simulink library "momentum_flight_control_v1"  (R2022a)
settings: Solver=VariableStepAuto  StartTime=0.0  StopTime=10.0  RelTol=1e-3
undefined symbols (not defined in the file): biasVectorConstraint_feet, Config, ConstraintMatrix_feet, DiscIntNeverNeededParam, Frames
libraries: WBToolboxLibrary x40
(part 2 of 2)

== system momentum_flight_control_v1/Flight Controller RAL-HUMANOIDS V3.0/Joint Torque Control for Flying/QP torqueControl/QP torqueControl - balancing ==
  H : Inport
  g : Inport  Port=2
  ub : Inport  Port=3
  lb : Inport  Port=4
  AEq : Inport  Port=5
  lbEq : Inport  Port=6
  ubEq : Inport  Port=7
  Enable : EnablePort
  Combine Bounds and Inequalities : MATLAB Function  TreatAsAtomicUnit=on
  MatchSignalSizes : WBToolboxLibrary/Utilities/MatchSignalSizes
      settings: SourceProductName=WholeBodyToolbox
  QP balancing-torqueControl : WBToolboxLibrary/Utilities/QP  lbA=on  ubA=on  lb=off  ub=off  computeObjVal=off  stopIfFails=off
      settings: SourceProductName=WholeBodyToolbox
  QPStatus_balancing : Outport  VectorParamsAs1DForOutWhenUnconnected=off
  QPOutput_balancing : Outport  Port=2  VectorParamsAs1DForOutWhenUnconnected=off
  wires:
  QP balancing-torqueControl/2 -> QPStatus_balancing/1
  MatchSignalSizes/1 -> QPOutput_balancing/1
  QP balancing-torqueControl/1 -> MatchSignalSizes/2
  H/1 -> QP balancing-torqueControl/1
  g/1 -> MatchSignalSizes/1, QP balancing-torqueControl/2
  AEq/1 -> Combine Bounds and Inequalities/1(AEq)
  lbEq/1 -> Combine Bounds and Inequalities/2(lbEq)
  ubEq/1 -> Combine Bounds and Inequalities/3(ubEq)
  lb/1 -> Combine Bounds and Inequalities/4(lb)
  ub/1 -> Combine Bounds and Inequalities/5(ub)
  Combine Bounds and Inequalities/1(AEq_combined) -> QP balancing-torqueControl/3
  Combine Bounds and Inequalities/2(lbEq_combined) -> QP balancing-torqueControl/4
  Combine Bounds and Inequalities/3(ubEq_combined) -> QP balancing-torqueControl/5

== system momentum_flight_control_v1/Flight Controller RAL-HUMANOIDS V3.0/Joint Torque Control for Flying/QP torqueControl/QP torqueControl - flight ==
  H : Inport
  g : Inport  Port=2
  ub : Inport  Port=3
  lb : Inport  Port=4
  Enable : EnablePort
  MatchSignalSizes : WBToolboxLibrary/Utilities/MatchSignalSizes
      settings: SourceProductName=WholeBodyToolbox
  QP flight-torqueControl : WBToolboxLibrary/Utilities/QP  lbA=off  ubA=off  lb=on  ub=on  computeObjVal=off  stopIfFails=off
      settings: SourceProductName=WholeBodyToolbox
  QPStatus_flight : Outport  VectorParamsAs1DForOutWhenUnconnected=off
  QPOutput_flight : Outport  Port=2  VectorParamsAs1DForOutWhenUnconnected=off
  wires:
  QP flight-torqueControl/2 -> QPStatus_flight/1
  lb/1 -> QP flight-torqueControl/3
  MatchSignalSizes/1 -> QPOutput_flight/1
  QP flight-torqueControl/1 -> MatchSignalSizes/2
  H/1 -> QP flight-torqueControl/1
  g/1 -> QP flight-torqueControl/2, MatchSignalSizes/1
  ub/1 -> QP flight-torqueControl/4

== system momentum_flight_control_v1/Flight Controller RAL-HUMANOIDS V3.0/Joint Torque Control for Flying/QP torqueControl/Select QP torqueControl Output ==
  QPStatus_balancing : Inport
  QPOutput_balancing : Inport  Port=2
  feetContactIsActive : Inport  Port=3
  QPStatus_flight : Inport  Port=4
  QPOutput_flight : Inport  Port=5
  Demux : Demux  Outputs=[12;Config.N_DOF]
  Switch : Switch  Criteria=u2 > Threshold  SaturateOnIntegerOverflow=off  InputSameDT=off
  Switch1 : Switch  Criteria=u2 > Threshold  SaturateOnIntegerOverflow=off  InputSameDT=off
  contactForces_QP : Terminator
  jointTorques_star : Outport  VectorParamsAs1DForOutWhenUnconnected=off
  exitFlagQP_torqueControl : Outport  Port=2  VectorParamsAs1DForOutWhenUnconnected=off
  wires:
  Switch1/1 -> jointTorques_star/1
  feetContactIsActive/1 -> Switch1/2, Switch/2
  QPStatus_balancing/1 -> Switch/1
  QPStatus_flight/1 -> Switch/3
  Switch/1 -> exitFlagQP_torqueControl/1
  QPOutput_balancing/1 -> Demux/1
  QPOutput_flight/1 -> Switch1/3
  Demux/1 -> contactForces_QP/1
  Demux/2 -> Switch1/1

== system momentum_flight_control_v1/Flight Controller RAL-HUMANOIDS V3.0/Momentum Control for Flying/QP Solver and Integrate Contact Forces Derivative/Integrate the Contact Forces Derivative ==
  contactForcesDot_star : Inport
  contactForces : Inport  Port=2
  feetContactIsActive : Inport  Port=3
  Discrete-Time Integrator1 : DiscreteIntegrator  ExternalReset=either  InitialConditionSource=external  InitialCondition=zeros(6,1)  SampleTime=Config.tStep  ICPrevOutput=DiscIntNeverNeededParam  ICPrevScaledInput=DiscIntNeverNeededParam
  Select Integrator Initial Condition : MATLAB Function  TreatAsAtomicUnit=on
  deadZone : Subsystem
  contactForces_star : Outport  VectorParamsAs1DForOutWhenUnconnected=off
  tag scope: contactForcesDot_star=global
  wires:
  Discrete-Time Integrator1/1 -> contactForces_star/1
  contactForcesDot_star/1 -> deadZone/1(u), [contactForcesDot_star]
  deadZone/1(u_cut) -> Discrete-Time Integrator1/1
  contactForces/1 -> Select Integrator Initial Condition/2(contactForces)
  feetContactIsActive/1 -> Select Integrator Initial Condition/1(feetContactIsActive), Discrete-Time Integrator1/2
  Select Integrator Initial Condition/1(contactForces_0) -> Discrete-Time Integrator1/3

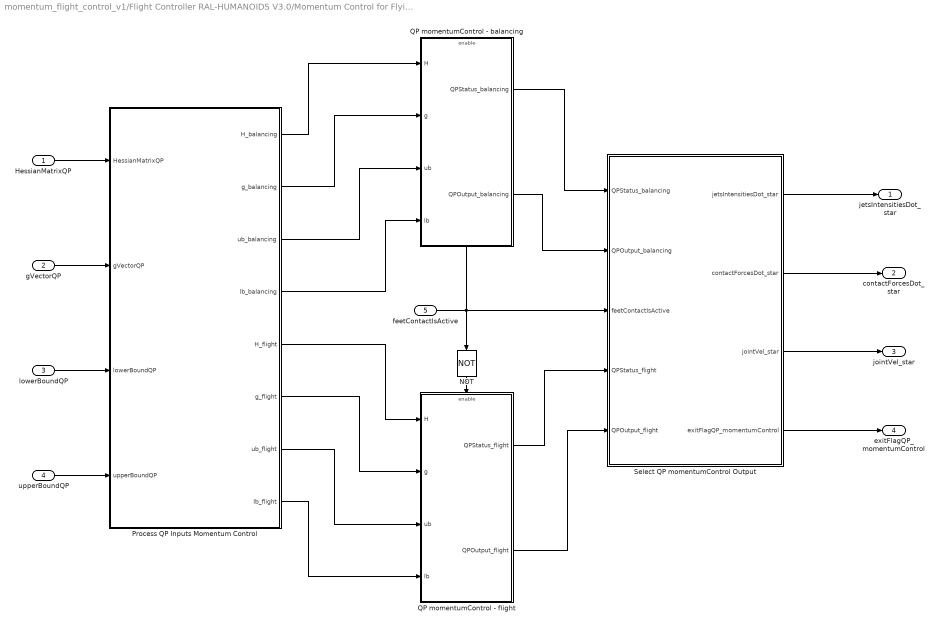
== system momentum_flight_control_v1/Flight Controller RAL-HUMANOIDS V3.0/Momentum Control for Flying/QP Solver and Integrate Contact Forces Derivative/QP momentumControl ==
  HessianMatrixQP : Inport
  gVectorQP : Inport  Port=2
  lowerBoundQP : Inport  Port=3
  upperBoundQP : Inport  Port=4
  feetContactIsActive : Inport  Port=5
  NOT : Logic  Operator=NOT  IconShape=distinctive  AllPortsSameDT=off  OutDataTypeStr=boolean
  Process QP Inputs Momentum Control : MATLAB Function  TreatAsAtomicUnit=on
  QP momentumControl - balancing : Subsystem  TreatAsAtomicUnit=on
  QP momentumControl - flight : Subsystem  TreatAsAtomicUnit=on
  Select QP momentumControl Output : Subsystem
  jetsIntensitiesDot_star : Outport  VectorParamsAs1DForOutWhenUnconnected=off
  contactForcesDot_star : Outport  Port=2  VectorParamsAs1DForOutWhenUnconnected=off
  jointVel_star : Outport  Port=3  VectorParamsAs1DForOutWhenUnconnected=off
  exitFlagQP_momentumControl : Outport  Port=4  VectorParamsAs1DForOutWhenUnconnected=off
  wires:
  gVectorQP/1 -> Process QP Inputs Momentum Control/2(gVectorQP)
  lowerBoundQP/1 -> Process QP Inputs Momentum Control/3(lowerBoundQP)
  feetContactIsActive/1 -> Select QP momentumControl Output/3(feetContactIsActive), NOT/1, QP momentumControl - balancing/Enable
  upperBoundQP/1 -> Process QP Inputs Momentum Control/4(upperBoundQP)
  HessianMatrixQP/1 -> Process QP Inputs Momentum Control/1(HessianMatrixQP)
  Select QP momentumControl Output/1(jetsIntensitiesDot_star) -> jetsIntensitiesDot_star/1
  Select QP momentumControl Output/3(jointVel_star) -> jointVel_star/1
  Select QP momentumControl Output/2(contactForcesDot_star) -> contactForcesDot_star/1
  Process QP Inputs Momentum Control/1(H_balancing) -> QP momentumControl - balancing/1(H)
  Process QP Inputs Momentum Control/2(g_balancing) -> QP momentumControl - balancing/2(g)
  Process QP Inputs Momentum Control/5(H_flight) -> QP momentumControl - flight/1(H)
  Process QP Inputs Momentum Control/6(g_flight) -> QP momentumControl - flight/2(g)
  Process QP Inputs Momentum Control/3(ub_balancing) -> QP momentumControl - balancing/3(ub)
  Process QP Inputs Momentum Control/4(lb_balancing) -> QP momentumControl - balancing/4(lb)
  Process QP Inputs Momentum Control/7(ub_flight) -> QP momentumControl - flight/3(ub)
  Process QP Inputs Momentum Control/8(lb_flight) -> QP momentumControl - flight/4(lb)
  NOT/1 -> QP momentumControl - flight/Enable
  Select QP momentumControl Output/4(exitFlagQP_momentumControl) -> exitFlagQP_momentumControl/1
  QP momentumControl - balancing/1(QPStatus_balancing) -> Select QP momentumControl Output/1(QPStatus_balancing)
  QP momentumControl - balancing/2(QPOutput_balancing) -> Select QP momentumControl Output/2(QPOutput_balancing)
  QP momentumControl - flight/1(QPStatus_flight) -> Select QP momentumControl Output/4(QPStatus_flight)
  QP momentumControl - flight/2(QPOutput_flight) -> Select QP momentumControl Output/5(QPOutput_flight)

== system momentum_flight_control_v1/Flight State Machine/Compute Gains And References/Smooth CoM and Base References/Smooth Position References ==
  smoothingTimeCoMPos : Inport
  pos_vel_acc_jerk_CoM_des : Inport  Port=2
  "CoM6D -> CoMXYZ5" : Selector  NumberOfDimensions=2  InputPortWidth=7  IndexOptions=Index vector (dialog),Index vector (dialog)  Indices=[1 2 3],[1]  OutputSizes=1,1
  Compute Smooth Jerk Reference : WBToolboxLibrary/Utilities/MinimumJerkTrajectoryGenerator  externalSettlingTime=off  settlingTime=Config.references.com.tSmoothingCoMAcc  sampleTime=Config.tStep  resetOnSettlingTime=off  firstDerivatives=on  secondDerivatives=off  explicitInitialValue=off
      settings: SourceProductName=WholeBodyToolbox
  Matrix Concatenate : Concatenate  NumInputs=4  Mode=Multidimensional array  ConcatenateDimension=2
  MinimumJerkTrajectoryGenerator : WBToolboxLibrary/Utilities/MinimumJerkTrajectoryGenerator  externalSettlingTime=on  settlingTime=3  sampleTime=Config.tStep  resetOnSettlingTime=off  firstDerivatives=on  secondDerivatives=on  explicitInitialValue=off
      settings: SourceProductName=WholeBodyToolbox
  Terminator : Terminator
  pos_vel_acc_jerk_CoM_des_smooth : Outport  VectorParamsAs1DForOutWhenUnconnected=off
  wires:
  pos_vel_acc_jerk_CoM_des/1 -> "CoM6D -> CoMXYZ5"/1
  smoothingTimeCoMPos/1 -> MinimumJerkTrajectoryGenerator/2
  MinimumJerkTrajectoryGenerator/1 -> Matrix Concatenate/1
  Matrix Concatenate/1 -> pos_vel_acc_jerk_CoM_des_smooth/1
  "CoM6D -> CoMXYZ5"/1 -> MinimumJerkTrajectoryGenerator/1
  MinimumJerkTrajectoryGenerator/2 -> Matrix Concatenate/2
  MinimumJerkTrajectoryGenerator/3 -> Matrix Concatenate/3, Compute Smooth Jerk Reference/1
  Compute Smooth Jerk Reference/1 -> Terminator/1
  Compute Smooth Jerk Reference/2 -> Matrix Concatenate/4

== system momentum_flight_control_v1/Flight State Machine/Compute Gains And References/Smooth CoM and Base References/Smooth Reference Orientations ==
  rot_vel_acc_jerk_base_des : Inport
  gainSmoothingBaseRot : Inport  Port=2
  Matrix Concatenate6 : Concatenate  NumInputs=4  Mode=Multidimensional array  ConcatenateDimension=2
  MinimumJerkTrajectoryGenerator : WBToolboxLibrary/Utilities/MinimumJerkTrajectoryGenerator  externalSettlingTime=off  settlingTime=Config.references.orientation.tSmoothingAngVel  sampleTime=Config.tStep  resetOnSettlingTime=off  firstDerivatives=on  secondDerivatives=on  explicitInitialValue=off
      settings: SourceProductName=WholeBodyToolbox
  Rotational PID Controller : Subsystem
  Selector : Selector  NumberOfDimensions=2  InputPortWidth=3  IndexOptions=Index vector (dialog),Index vector (dialog)  Indices=[1:3],[1:3]  OutputSizes=1,1
  rot_acc_vel_jerk_base_des_smooth : Outport  VectorParamsAs1DForOutWhenUnconnected=off
  wires:
  rot_vel_acc_jerk_base_des/1 -> Selector/1
  Matrix Concatenate6/1 -> rot_acc_vel_jerk_base_des_smooth/1
  Rotational PID Controller/1(w_R_b_des_smooth) -> Matrix Concatenate6/1
  Rotational PID Controller/2(body_omega_b_des_smooth) -> MinimumJerkTrajectoryGenerator/1
  MinimumJerkTrajectoryGenerator/1 -> Matrix Concatenate6/2
  MinimumJerkTrajectoryGenerator/2 -> Matrix Concatenate6/3
  Selector/1 -> Rotational PID Controller/1(w_R_b_des)
  gainSmoothingBaseRot/1 -> Rotational PID Controller/2(gainSmoothingBaseRot)
  MinimumJerkTrajectoryGenerator/3 -> Matrix Concatenate6/4

== system momentum_flight_control_v1/Flight Controller RAL-HUMANOIDS V3.0/Momentum Control for Flying/QP Solver and Integrate Contact Forces Derivative/Integrate the Contact Forces Derivative/deadZone ==
  u : Inport
  Constant : Constant  Value=Config.sat.deadZoneThreshold
  Deadzone Function : MATLAB Function  TreatAsAtomicUnit=on
  u_cut : Outport  VectorParamsAs1DForOutWhenUnconnected=off
  wires:
  Deadzone Function/1(y) -> u_cut/1
  u/1 -> Deadzone Function/1(u)
  Constant/1 -> Deadzone Function/2(thr)

== system momentum_flight_control_v1/Flight Controller RAL-HUMANOIDS V3.0/Momentum Control for Flying/QP Solver and Integrate Contact Forces Derivative/QP momentumControl/QP momentumControl - balancing ==
  H : Inport
  g : Inport  Port=2
  ub : Inport  Port=3
  lb : Inport  Port=4
  Enable : EnablePort
  MatchSignalSizes : WBToolboxLibrary/Utilities/MatchSignalSizes
      settings: SourceProductName=WholeBodyToolbox
  QP balancing-momentumControl : WBToolboxLibrary/Utilities/QP  lbA=off  ubA=off  lb=on  ub=on  computeObjVal=off  stopIfFails=off
      settings: SourceProductName=WholeBodyToolbox
  QPStatus_balancing : Outport  VectorParamsAs1DForOutWhenUnconnected=off
  QPOutput_balancing : Outport  Port=2  VectorParamsAs1DForOutWhenUnconnected=off
  wires:
  QP balancing-momentumControl/2 -> QPStatus_balancing/1
  lb/1 -> QP balancing-momentumControl/3
  MatchSignalSizes/1 -> QPOutput_balancing/1
  QP balancing-momentumControl/1 -> MatchSignalSizes/2
  H/1 -> QP balancing-momentumControl/1
  g/1 -> QP balancing-momentumControl/2, MatchSignalSizes/1
  ub/1 -> QP balancing-momentumControl/4

== system momentum_flight_control_v1/Flight Controller RAL-HUMANOIDS V3.0/Momentum Control for Flying/QP Solver and Integrate Contact Forces Derivative/QP momentumControl/QP momentumControl - flight ==
  H : Inport
  g : Inport  Port=2
  ub : Inport  Port=3
  lb : Inport  Port=4
  Enable : EnablePort
  MatchSignalSizes : WBToolboxLibrary/Utilities/MatchSignalSizes
      settings: SourceProductName=WholeBodyToolbox
  QP flight-momentumControl : WBToolboxLibrary/Utilities/QP  lbA=off  ubA=off  lb=on  ub=on  computeObjVal=off  stopIfFails=off
      settings: SourceProductName=WholeBodyToolbox
  QPStatus_flight : Outport  VectorParamsAs1DForOutWhenUnconnected=off
  QPOutput_flight : Outport  Port=2  VectorParamsAs1DForOutWhenUnconnected=off
  wires:
  QP flight-momentumControl/2 -> QPStatus_flight/1
  lb/1 -> QP flight-momentumControl/3
  MatchSignalSizes/1 -> QPOutput_flight/1
  QP flight-momentumControl/1 -> MatchSignalSizes/2
  H/1 -> QP flight-momentumControl/1
  g/1 -> QP flight-momentumControl/2, MatchSignalSizes/1
  ub/1 -> QP flight-momentumControl/4

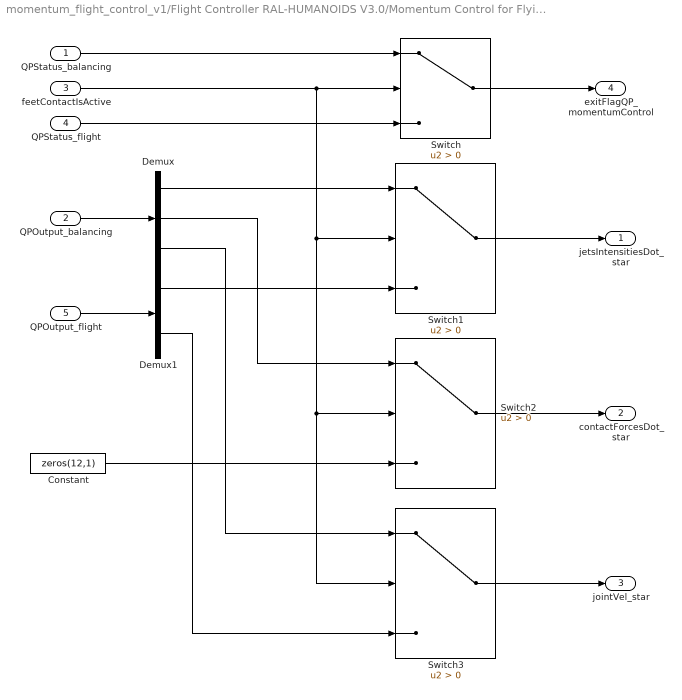
== system momentum_flight_control_v1/Flight Controller RAL-HUMANOIDS V3.0/Momentum Control for Flying/QP Solver and Integrate Contact Forces Derivative/QP momentumControl/Select QP momentumControl Output ==
  QPStatus_balancing : Inport
  QPOutput_balancing : Inport  Port=2
  feetContactIsActive : Inport  Port=3
  QPStatus_flight : Inport  Port=4
  QPOutput_flight : Inport  Port=5
  Constant : Constant  Value=zeros(12,1)
  Demux : Demux  Outputs=[4;12;Config.N_DOF]
  Demux1 : Demux  Outputs=[4;Config.N_DOF]
  Switch{,1..3} (4 alike) : Switch  Criteria=u2 > Threshold  SaturateOnIntegerOverflow=off  InputSameDT=off
  jetsIntensitiesDot_star : Outport  VectorParamsAs1DForOutWhenUnconnected=off
  contactForcesDot_star : Outport  Port=2  VectorParamsAs1DForOutWhenUnconnected=off
  jointVel_star : Outport  Port=3  VectorParamsAs1DForOutWhenUnconnected=off
  exitFlagQP_momentumControl : Outport  Port=4  VectorParamsAs1DForOutWhenUnconnected=off
  wires:
  Switch2/1 -> contactForcesDot_star/1
  Switch1/1 -> jetsIntensitiesDot_star/1
  Switch3/1 -> jointVel_star/1
  feetContactIsActive/1 -> Switch3/2, Switch2/2, Switch1/2, Switch/2
  QPStatus_balancing/1 -> Switch/1
  QPStatus_flight/1 -> Switch/3
  Switch/1 -> exitFlagQP_momentumControl/1
  QPOutput_balancing/1 -> Demux/1
  QPOutput_flight/1 -> Demux1/1
  Demux/1 -> Switch1/1
  Demux1/1 -> Switch1/3
  Demux/2 -> Switch2/1
  Constant/1 -> Switch2/3
  Demux/3 -> Switch3/1
  Demux1/2 -> Switch3/3

== system momentum_flight_control_v1/Flight State Machine/Compute Gains And References/Smooth CoM and Base References/Smooth Reference Orientations/Rotational PID Controller ==
  w_R_b_des : Inport
  gainSmoothingBaseRot : Inport  Port=2
  Compute Rotation Matrix Derivative : MATLAB Function  TreatAsAtomicUnit=on
  Discrete-Time Integrator2 : DiscreteIntegrator  InitialConditionSource=external  InitialCondition=zeros(3,1)  SampleTime=Config.tStep  ICPrevOutput=DiscIntNeverNeededParam  ICPrevScaledInput=DiscIntNeverNeededParam
  "holder " : WBToolboxLibrary/Utilities/holder 
      settings: SourceProductName=WholeBodyToolbox
  w_R_b_des_smooth : Outport  VectorParamsAs1DForOutWhenUnconnected=off
  body_omega_b_des_smooth : Outport  Port=2  VectorParamsAs1DForOutWhenUnconnected=off
  wires:
  "holder "/1 -> Discrete-Time Integrator2/2
  Compute Rotation Matrix Derivative/2(RDot) -> Discrete-Time Integrator2/1
  Discrete-Time Integrator2/1 -> w_R_b_des_smooth/1, Compute Rotation Matrix Derivative/3(w_R_b)
  w_R_b_des/1 -> "holder "/1, Compute Rotation Matrix Derivative/2(w_R_b_des)
  Compute Rotation Matrix Derivative/1(b_omega_b) -> body_omega_b_des_smooth/1
  gainSmoothingBaseRot/1 -> Compute Rotation Matrix Derivative/1(gainSmoothingBaseRot)

== matlab function momentum_flight_control_v1/Get System State/fromPosRPYtoTransfMatrix ==
  data: pos_rpy input; w_H_b output
function w_H_b = fromPosRpyToTransfMatrixFCN(pos_rpy)

    w_H_b = wbc.fromPosRpyToTransfMatrix(pos_rpy);
end

== matlab function momentum_flight_control_v1/Flight Controller RAL-HUMANOIDS V3.0/Joint Torque Control for Flying/QP torqueControl/Process QP Inputs Torque Control ==
  data: HessianMatrixQP input; H_balancing output; gVectorQP input; InequalityConstrMatrix input; biasVectorInequalityConstr input; g_balancing output; ub_balancing output; lb_balancing output; Aeq_balancing output; lbEq_balancing output; ubEq_balancing output; H_flight output; g_flight output; ub_flight output; lb_flight output; jointTorquesSaturation input; Config parameter
function [H_balancing,g_balancing,ub_balancing,lb_balancing,Aeq_balancing,lbEq_balancing,ubEq_balancing, ...
          H_flight,g_flight,ub_flight,lb_flight] = processQPinputTorqueControlFCN ...
                                                       (HessianMatrixQP,gVectorQP,InequalityConstrMatrix, ...
                                                        biasVectorInequalityConstr,jointTorquesSaturation,Config)   
   
[H_balancing,g_balancing,ub_balancing,lb_balancing,Aeq_balancing,lbEq_balancing,ubEq_balancing, ...
          H_flight,g_flight,ub_flight,lb_flight] = iRonCubLib_v1.processQPinputTorqueControl ...
                                                       (HessianMatrixQP,gVectorQP,InequalityConstrMatrix, ...
                                                        biasVectorInequalityConstr,jointTorquesSaturation,Config);     
end

== matlab function momentum_flight_control_v1/Flight Controller RAL-HUMANOIDS V3.0/Joint Torque Control for Flying/QP torqueControl/QP torqueControl - balancing/Combine Bounds and Inequalities ==
  data: AEq input; AEq_combined output; lbEq input; ubEq input; lb input; ub input; lbEq_combined output; ubEq_combined output
function [AEq_combined,lbEq_combined,ubEq_combined] = combineInputBoundsAndInequalitiesQPFCN(AEq,lbEq,ubEq,lb,ub)

   [AEq_combined,lbEq_combined,ubEq_combined] = iRonCubLib.combineInputBoundsAndInequalitiesQP(AEq,lbEq,ubEq,lb,ub);
end

== matlab function momentum_flight_control_v1/Dynamics and Kinematics/Dynamic Quantities/Compute Centroidal Inertia/Compute Centroidal Inertia ==
  data: M input; w_I_c output; posCoM input; posBase input
function w_I_c = getCentrInertiaFCN(M, posCoM, posBase)

    w_I_c = iRonCubLib_v1.getCentrInertia(M, posCoM, posBase);
end

== matlab function momentum_flight_control_v1/Flight State Machine/Take Off//Landing State Detector/MATLAB Function ==
  data: wrench_l input; feetContactIsActive output; wrench_r input; Config parameter; robotIsLanded output; oneFootIsInContact output
function [feetContactIsActive, robotIsLanded, oneFootIsInContact] = feetContactActivationFCN(wrench_l, wrench_r, Config)

    [feetContactIsActive, robotIsLanded, oneFootIsInContact] = iRonCubLib_v1.feetContactActivation(wrench_l, wrench_r, Config);
end

== matlab function momentum_flight_control_v1/Flight Controller RAL-HUMANOIDS V3.0/Joint Torque Control for Flying/Torque Derivative Saturation/Saturate Torque Derivative ==
  data: u input; uSat output; u_0 input; tStep input; uDotMax input
function uSat = saturateInputDerivativeFCN(u, u_0, tStep, uDotMax)

    uSat = wbc.saturateInputDerivative(u, u_0, tStep, uDotMax);
end

== matlab function momentum_flight_control_v1/JoyStick-flightGUI Commands/Replace Joystick with Native GUI ==
  data: gui_input input; joyButtons output; joyAxes output
function [joyButtons,joyAxes] = fromGuiToJoystickFCN(gui_input)

    [joyButtons,joyAxes] = iRonCubLib_v1.fromGuiToJoystick(gui_input);
end

== matlab function momentum_flight_control_v1/Get System State/Change Contact Forces Representation/Change Contact Forces Representation ==
  data: contactForces_WBD input; mixed_f_l_sole output; w_R_l_sole input; w_R_r_sole input; mixed_f_r_sole output
function [mixed_f_l_sole,mixed_f_r_sole] = fromBodyFrameToMixed_contactForcesFCN(contactForces_WBD,w_R_l_sole,w_R_r_sole)

    [mixed_f_l_sole,mixed_f_r_sole] = iRonCubLib_v1.fromBodyFrameToMixed_contactForces(contactForces_WBD,w_R_l_sole,w_R_r_sole);
end

== matlab function momentum_flight_control_v1/Flight State Machine/Compute Gains And References/Compute Gains/Diagonalize ==
  data: k input; K output
function K = diagonalMatrixFromVectorFCN(k)

    K = wbc.diagonalMatrixFromVector(k);
end

== matlab function momentum_flight_control_v1/Flight State Machine/Compute Gains And References/Compute Gains/Diagonalize1 ==
  data: k input; K output
function K = diagonalMatrixFromVectorFCN(k)

    K = wbc.diagonalMatrixFromVector(k);
end

== matlab function momentum_flight_control_v1/Flight State Machine/Compute Gains And References/Compute Gains/Diagonalize2 ==
  data: k input; K output
function K = diagonalMatrixFromVectorFCN(k)

    K = wbc.diagonalMatrixFromVector(k);
end

== matlab function momentum_flight_control_v1/Flight Controller RAL-HUMANOIDS V3.0/Momentum Control for Flying/Momentum Control/Flying Controller Momentum FCN  ==
  data: jointPos input; w_baseTwist input; jetsIntensities input; J_jets input; J_CoM input; J_LFoot input; J_RFoot input; posCoM input; w_R_b input; w_H_LFoot input; w_H_RFoot input; matrixOfJetsAxes input; matrixOfJetsArms input; w_I_c input; L input; M input; CMM input; pos_vel_acc_jerk_CoM_des input; rot_vel_acc_jerk_base_des input size=[3,6]; jointPos_des input; KP_momentum input; KD_momentum input; KP_postural input; feetContactIsActive input; decreaseMaxFootVerticalForce input; increaseMinFootVerticalForce input; robotIsLanded input; HessianMatrixQP output; gVectorQP output; lowerBoundQP output; upperBoundQP output; L_des output; LDot_estimated output; verifyAngMomAndInertia output; contactForces_hat input; Config parameter; velCoM output
function [HessianMatrixQP, gVectorQP, lowerBoundQP, upperBoundQP, L_des, LDot_estimated, verifyAngMomAndInertia, velCoM] = ...
             flyingMomentumControlFCN(jointPos, w_baseTwist, jetsIntensities, J_jets, J_CoM, J_LFoot, J_RFoot, posCoM, w_R_b, w_H_LFoot, ...
                                      w_H_RFoot, matrixOfJetsAxes, matrixOfJetsArms, w_I_c, L, M, CMM, pos_vel_acc_jerk_CoM_des, ....
                                      rot_vel_acc_jerk_base_des, jointPos_des, KP_momentum, KD_momentum, KP_postural, feetContactIsActive, ...
                                      decreaseMaxFootVerticalForce, increaseMinFootVerticalForce, robotIsLanded, contactForces_hat, Config)
                               
    [HessianMatrixQP, gVectorQP, lowerBoundQP, upperBoundQP, L_des, LDot_estimated, verifyAngMomAndInertia, velCoM] = ...
        iRonCubLib_v1.flyingMomentumControl(jointPos, w_baseTwist, jetsIntensities, J_jets, J_CoM, J_LFoot, J_RFoot, posCoM, w_R_b, w_H_LFoot, ...
                                            w_H_RFoot, matrixOfJetsAxes, matrixOfJetsArms, w_I_c, L, M, CMM, pos_vel_acc_jerk_CoM_des, ....
                                            rot_vel_acc_jerk_base_des, jointPos_des, KP_momentum, KD_momentum, KP_postural, feetContactIsActive, ...
                                            decreaseMaxFootVerticalForce, increaseMinFootVerticalForce, robotIsLanded, contactForces_hat, Config);
end

== matlab function momentum_flight_control_v1/Flight Controller RAL-HUMANOIDS V3.0/Joint Torque Control for Flying/torqueControlFCN ==
  data: M input; h input; J_jets input; J_LFoot input; J_RFoot input; JDot_LFoot_nu input; JDot_RFoot_nu input; w_H_LFoot input; w_H_RFoot input; matrixOfJetsAxes input; ConstraintsMatrix_feet input; biasVectorConstraint_feet input; jetsIntensities input; stateVel input; jointVel_star input; contactForces_star input; KI_torqueControl input; KP_torqueControl input; feetContactIsActive input; activateEqConstrTorqueControl input; robotIsLanded input; jointPos_err input; Hessian output; Config parameter; gradient output; ConstraintMatrix_inequality output; biasVectorConstraint_inequality output; jointVel_err output
function [Hessian, gradient, ConstraintMatrix_inequality, biasVectorConstraint_inequality, jointVel_err] =  ... 
             flyingTorqueControlFCN(M, h, J_jets, J_LFoot, J_RFoot, JDot_LFoot_nu, JDot_RFoot_nu, w_H_LFoot, w_H_RFoot, matrixOfJetsAxes, ...
                                    ConstraintsMatrix_feet, biasVectorConstraint_feet, jetsIntensities, stateVel, jointVel_star, contactForces_star, ...
                                    KI_torqueControl, KP_torqueControl, feetContactIsActive, activateEqConstrTorqueControl, robotIsLanded, jointPos_err, Config)
                                      
    [Hessian, gradient, ConstraintMatrix_inequality, biasVectorConstraint_inequality, jointVel_err] =  ... 
        iRonCubLib_v1.flyingTorqueControl(M, h, J_jets, J_LFoot, J_RFoot, JDot_LFoot_nu, JDot_RFoot_nu, w_H_LFoot, w_H_RFoot, matrixOfJetsAxes, ...
                                          ConstraintsMatrix_feet, biasVectorConstraint_feet, jetsIntensities, stateVel, jointVel_star, contactForces_star, ...
                                          KI_torqueControl, KP_torqueControl, feetContactIsActive, activateEqConstrTorqueControl, robotIsLanded, jointPos_err, Config);           
end

== matlab function momentum_flight_control_v1/Flight State Machine/Compute Gains And References/Compute Gains/Diagonalize3 ==
  data: k input; K output
function K = diagonalMatrixFromVectorFCN(k)

    K = wbc.diagonalMatrixFromVector(k);
end

== matlab function momentum_flight_control_v1/Dynamics and Kinematics/Kinematic Quantities/Compute Thrusts Axes and Arms/Thrust Axes and Arms ==
  data: w_H_J1 input; matrixOfJetsAxes output; w_H_J2 input; w_H_J3 input; w_H_J4 input; posCoM input; matrixOfJetsArms output; Config parameter
function [matrixOfJetsAxes, matrixOfJetsArms] = computeJetsAxesAndArmsFCN(w_H_J1, w_H_J2, w_H_J3, w_H_J4, posCoM, Config)

    [matrixOfJetsAxes, matrixOfJetsArms] = iRonCubLib_v1.computeJetsAxesAndArms(w_H_J1, w_H_J2, w_H_J3, w_H_J4, posCoM, Config);
end

== matlab function momentum_flight_control_v1/Flight State Machine/Compute Gains And References/Compute Gains/Diagonalize4 ==
  data: k input; K output
function K = diagonalMatrixFromVectorFCN(k)

    K = wbc.diagonalMatrixFromVector(k);
end

== matlab function momentum_flight_control_v1/Flight Controller RAL-HUMANOIDS V3.0/Momentum Control for Flying/QP Solver and Integrate Contact Forces Derivative/Integrate the Contact Forces Derivative/deadZone/Deadzone Function ==
  data: u input; y output; thr input
function y = deadZoneFCN(u, thr)

    y = wbc.deadZone(u, thr);
end

== matlab function momentum_flight_control_v1/Flight State Machine/Take Off//Landing State Detector/Vertical Forces Control ==
  data: joyButtons input; decreaseMaxFootVerticalForce output; increaseMinFootVerticalForce output; activateEqConstrTorqueControl output
function [decreaseMaxFootVerticalForce, increaseMinFootVerticalForce, activateEqConstrTorqueControl] = verticalForcesControlFCN(joyButtons)

    [decreaseMaxFootVerticalForce, increaseMinFootVerticalForce, activateEqConstrTorqueControl] = iRonCubLib_v1.verticalForcesControl(joyButtons);
end

== matlab function momentum_flight_control_v1/Flight Controller RAL-HUMANOIDS V3.0/Momentum Control for Flying/QP Solver and Integrate Contact Forces Derivative/Integrate the Contact Forces Derivative/Select Integrator Initial Condition ==
  data: feetContactIsActive input; contactForces input; contactForces_0 output
function contactForces_0 = selectInitContactForcesFCN(feetContactIsActive, contactForces)

    contactForces_0 = iRonCubLib.selectInitContactForces(feetContactIsActive, contactForces);
end

== matlab function momentum_flight_control_v1/Compute Fuel Consumption/Get the Current Fuel Consumption ==
  data: thrusts input; fuelConsCurr output; Config parameter
function fuelConsCurr = computeCurrentFuelConsumptionFCN(thrusts, Config)

    fuelConsCurr = iRonCubLib_v1.computeCurrentFuelConsumption(thrusts, Config);
end

== matlab function momentum_flight_control_v1/Flight State Machine/Compute Gains And References/Trajectory Generator/Compute CoM and Base Rotation References ==
  data: posCoM_init input; w_R_b_init input; moveFront input; pos_vel_acc_jerk_CoM_des output; moveLateral input; moveUpDown input; rotateRoll input; rotatePitch input; rotateYaw input; turbo_mode input; goLandingPos input; feetContactIsActive input; oneFootIsInContact input; t input; Config parameter; rot_vel_acc_jerk_base_des output
function [pos_vel_acc_jerk_CoM_des, rot_vel_acc_jerk_base_des] = ...
             computeReferencesBaseAndCoMFCN(posCoM_init, w_R_b_init, moveFront, moveLateral, moveUpDown, rotateRoll, rotatePitch, ...
                                            rotateYaw, turbo_mode, goLandingPos, feetContactIsActive, oneFootIsInContact, t, Config)
                                     
    [pos_vel_acc_jerk_CoM_des, rot_vel_acc_jerk_base_des] = ...
        iRonCubLib_v1.computeReferencesBaseAndCoM(posCoM_init, w_R_b_init, moveFront, moveLateral, moveUpDown, rotateRoll, rotatePitch, ...
                                                  rotateYaw, turbo_mode, goLandingPos, feetContactIsActive, oneFootIsInContact, t, Config);
end

== matlab function momentum_flight_control_v1/Flight State Machine/Compute Gains And References/Trajectory Generator/Detect Robot Movement Request From Joystick ==
  data: joyAxes input; moveFront output; moveLateral output; moveUpDown output; rotateRoll output; rotatePitch output; joyButtons input; rotateYaw output; turbo_mode output; goLandingPos output
function [moveFront,moveLateral,moveUpDown,rotateRoll,rotatePitch,rotateYaw,turbo_mode,goLandingPos] = detectMovementsFromJoystickFCN(joyAxes,joyButtons)

    [moveFront,moveLateral,moveUpDown,rotateRoll,rotatePitch,rotateYaw,turbo_mode,goLandingPos] = iRonCubLib_v1.detectMovementsFromJoystick(joyAxes,joyButtons);
end

== matlab function momentum_flight_control_v1/Flight State Machine/Compute Gains And References/Smooth CoM and Base References/Smooth Reference Orientations/Rotational PID Controller/Compute Rotation Matrix Derivative ==
  data: gainSmoothingBaseRot input; w_R_b_des input; w_R_b input; b_omega_b output; RDot output
function [b_omega_b, RDot] = rotationDerivativeFromAngVelFCN(gainSmoothingBaseRot, w_R_b_des, w_R_b)
                                                                                                                                                            
    % Rotational PID: 
    %
    % w_R_b_des = reference rotation (may be discontinuous)
    % 
    % b_omega_b = control input for the rotational PID. The angular velocity
    %             is expressed w.r.t. a frame attached to the link, i.e. it 
    %             is expressed in the "body" frame (b).
    % 
    % Kp        = control gain
    %
    % w_R_b     = smooth base rotation
    %
    b_omega_b_des       = zeros(3,1);
    Kp                  = gainSmoothingBaseRot;
    b_omega_b           = wbc.rotationalPID_bodyVelocity(w_R_b, w_R_b_des, b_omega_b_des, Kp);
                      
    % compute the rotation matrix derivative given the angular velocity in body frame
    RDot                = wbc.rotationDerivativeFromBodyAngVel(b_omega_b, w_R_b); 
end

== matlab function momentum_flight_control_v1/Flight Controller RAL-HUMANOIDS V3.0/Momentum Control for Flying/QP Solver and Integrate Contact Forces Derivative/QP momentumControl/Process QP Inputs Momentum Control ==
  data: HessianMatrixQP input; H_balancing output; gVectorQP input; lowerBoundQP input; upperBoundQP input; g_balancing output; ub_balancing output; lb_balancing output; H_flight output; g_flight output; ub_flight output; lb_flight output
function [H_balancing,g_balancing,ub_balancing,lb_balancing, ...
          H_flight,g_flight,ub_flight,lb_flight] = processQPinputMomentumControlFCN(HessianMatrixQP,gVectorQP,lowerBoundQP,upperBoundQP) 
      
    [H_balancing,g_balancing,ub_balancing,lb_balancing, ...
        H_flight,g_flight,ub_flight,lb_flight] = iRonCubLib_v1.processQPinputMomentumControl(HessianMatrixQP,gVectorQP,lowerBoundQP,upperBoundQP);
end
